simulink model "model_template"  (R2023b)
settings: Solver=VariableStepAuto  StartTime=0.0  StopTime=10.0  RelTol=1e-3
settings Model: Creator=bglen  LastModifiedBy=bglen

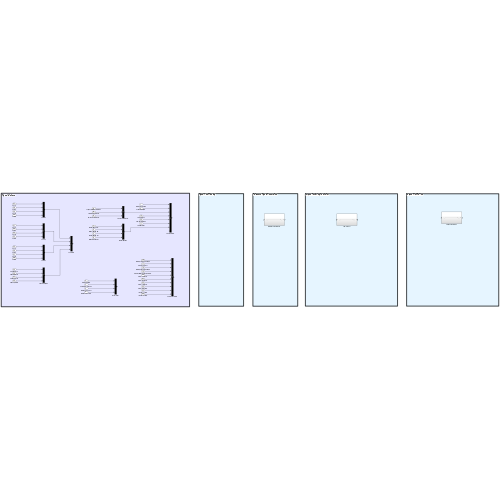
[thumbnail: Simulink's stored preview of the top-level diagram]
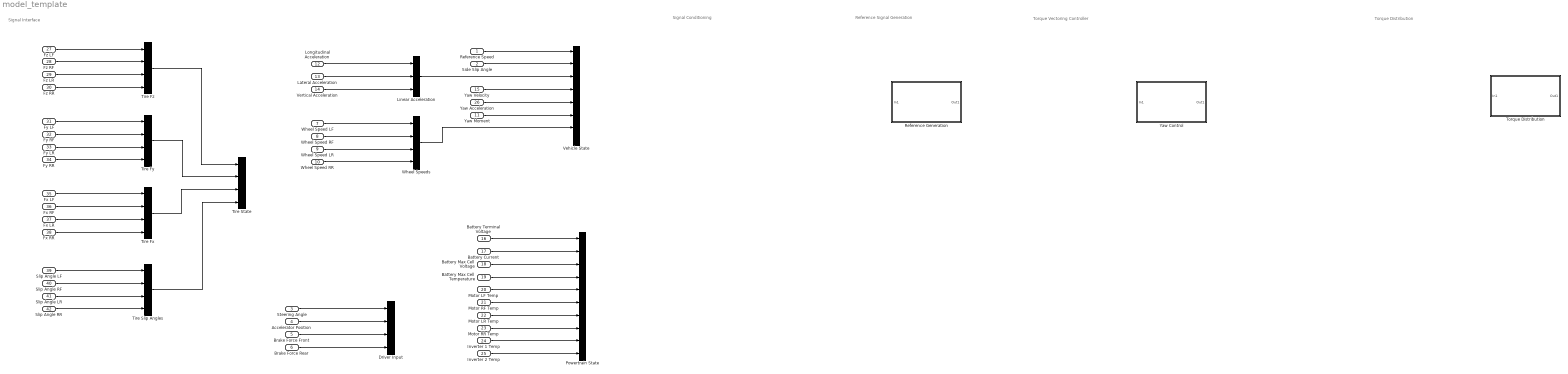
== system model_template ==
  note: Reference Signal Generation
  note: Torque Vectoring Controller
  note: Torque Distribution
  note: Signal Interface
  note: Signal Conditioning
  Reference Speed : Inport
  Side Slip Angle : Inport  Port=2
  Steering Angle : Inport  Port=3
  Accelerator Position : Inport  Port=4
  Brake Force Front : Inport  Port=5
  Brake Force Rear : Inport  Port=6
  Wheel Speed LF : Inport  Port=7
  Wheel Speed RF : Inport  Port=8
  Wheel Speed LR : Inport  Port=9
  Wheel Speed RR : Inport  Port=10
  Yaw Moment : Inport  Port=11
  Longitudinal Acceleration : Inport  Port=12
  Lateral Acceleration : Inport  Port=13
  Vertical Acceleration : Inport  Port=14
  Yaw Velocity : Inport  Port=15
  Battery Terminal Voltage : Inport  Port=16
  Battery Current : Inport  Port=17
  Battery Max Cell Voltage : Inport  Port=18
  Battery Max Cell Temperature : Inport  Port=19
  Motor LF Temp : Inport  Port=20
  Motor RF Temp : Inport  Port=21
  Motor LR Temp : Inport  Port=22
  Motor RR Temp : Inport  Port=23
  Inverter 1 Temp : Inport  Port=24
  Inverter 2 Temp : Inport  Port=25
  Yaw Acceleration : Inport  Port=26
  Fz LF : Inport  Port=27
  Fz RF : Inport  Port=28
  Fz LR : Inport  Port=29
  Fz RR : Inport  Port=30
  Fy LF : Inport  Port=31
  Fy RF : Inport  Port=32
  Fy LR : Inport  Port=33
  Fy RR : Inport  Port=34
  Fx LF : Inport  Port=35
  Fx RF : Inport  Port=36
  Fx LR : Inport  Port=37
  Fx RR : Inport  Port=38
  Slip Angle LF : Inport  Port=39
  Slip Angle RF : Inport  Port=40
  Slip Angle LR : Inport  Port=41
  Slip Angle RR : Inport  Port=42
  Driver Input : BusCreator  Inputs=4
  Linear Acceleration : BusCreator  Inputs=3
  Powertrain State : BusCreator  Inputs=10
  Reference Generation : Subsystem
  Tire Fx : BusCreator  Inputs=4
  Tire Fy : BusCreator  Inputs=4
  Tire Fz : BusCreator  Inputs=4
  Tire Slip Angles : BusCreator  Inputs=4
  Tire State : BusCreator  Inputs=4
  Torque Distribution : Subsystem
  Vehicle State : BusCreator  Inputs=8
  Wheel Speeds : BusCreator  Inputs=4
  Yaw Control : Subsystem
  wires:
  Reference Speed/1 -> Vehicle State/1
  Side Slip Angle/1 -> Vehicle State/2
  Steering Angle/1 -> Driver Input/1
  Accelerator Position/1 -> Driver Input/2
  Brake Force Front/1 -> Driver Input/3
  Brake Force Rear/1 -> Driver Input/4
  Wheel Speed LF/1 -> Wheel Speeds/1
  Wheel Speed RF/1 -> Wheel Speeds/2
  Wheel Speed LR/1 -> Wheel Speeds/3
  Wheel Speed RR/1 -> Wheel Speeds/4
  Lateral Acceleration/1 -> Linear Acceleration/2
  Vertical Acceleration/1 -> Linear Acceleration/3
  Longitudinal Acceleration/1 -> Linear Acceleration/1
  Battery Current/1 -> Powertrain State/2
  Battery Max Cell Voltage/1 -> Powertrain State/3
  Battery Terminal Voltage/1 -> Powertrain State/1
  Battery Max Cell Temperature/1 -> Powertrain State/4
  Motor LF Temp/1 -> Powertrain State/5
  Motor RF Temp/1 -> Powertrain State/6
  Motor LR Temp/1 -> Powertrain State/7
  Motor RR Temp/1 -> Powertrain State/8
  Inverter 1 Temp/1 -> Powertrain State/9
  Inverter 2 Temp/1 -> Powertrain State/10
  Linear Acceleration/1 -> Vehicle State/3
  Yaw Velocity/1 -> Vehicle State/4
  Yaw Acceleration/1 -> Vehicle State/5
  Yaw Moment/1 -> Vehicle State/6
  Fz RF/1 -> Tire Fz/2
  Fz LF/1 -> Tire Fz/1
  Fz LR/1 -> Tire Fz/3
  Fz RR/1 -> Tire Fz/4
  Wheel Speeds/1 -> Vehicle State/7
  Fy RF/1 -> Tire Fy/2
  Fy LR/1 -> Tire Fy/3
  Fy LF/1 -> Tire Fy/1
  Fy RR/1 -> Tire Fy/4
  Fx RF/1 -> Tire Fx/2
  Fx LR/1 -> Tire Fx/3
  Fx LF/1 -> Tire Fx/1
  Fx RR/1 -> Tire Fx/4
  Slip Angle LF/1 -> Tire Slip Angles/1
  Slip Angle RF/1 -> Tire Slip Angles/2
  Slip Angle RR/1 -> Tire Slip Angles/4
  Slip Angle LR/1 -> Tire Slip Angles/3
  Tire Fz/1 -> Tire State/1
  Tire Fy/1 -> Tire State/2
  Tire Fx/1 -> Tire State/3
  Tire Slip Angles/1 -> Tire State/4

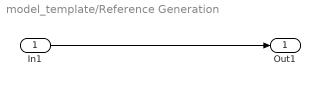
== system model_template/Reference Generation ==
  In1 : Inport
  Out1 : Outport
  wires:
  In1/1 -> Out1/1

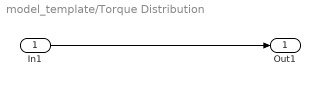
== system model_template/Torque Distribution ==
  In1 : Inport
  Out1 : Outport
  wires:
  In1/1 -> Out1/1

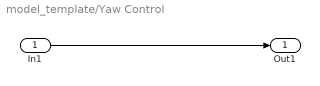
== system model_template/Yaw Control ==
  In1 : Inport
  Out1 : Outport
  wires:
  In1/1 -> Out1/1
